simulink model "QR_Unitree_with_spine"  (R2021b)
settings: Solver=ode23t  StartTime=0.0  StopTime=10  FixedStep=1e-2  MaxStep=0.01  RelTol=1e-3  AbsTol=1e-3  EnableMultiTasking=on
values from neighbouring files (symbols this model uses):
  body_dim = [0.267 0.194 0.114]    [last_scores.mat]    (also in robotParameters.m)
  body_mass = 6.0    (= 6)    [CostOfTransport.m]    (also in last_scores.mat; robotParameters.m)
  delta_gait_front = 48    [PD_optimizedData_16Mar22_1632.mat]    (also in PD_optimizedData_16Mar22_2228_good.mat = 58; PD_optimizedData_17Mar22_1432_vel_walk_03735.mat = 56; PD_optimizedData_18Mar22_1518_right_direction.mat = 46; PD_optimizedData_18Mar22_1539.mat = 88)
  delta_gait_rear = 56    [PD_optimizedData_16Mar22_1632.mat]    (also in PD_optimizedData_16Mar22_2228_good.mat = 40; PD_optimizedData_17Mar22_1432_vel_walk_03735.mat = 6; PD_optimizedData_18Mar22_1518_right_direction.mat = 76; PD_optimizedData_18Mar22_1539.mat = 42)
  fem_der_front = [0 1.0471975512 -3.66519142919 -6.45771823238 -0.523598775598 5.41052068118 0]    [last_scores.mat]
  fem_der_rear = [0 -2.61799387799 -0.872664625997 1.2217304764 4.88692190558 1.3962634016 0]    [last_scores.mat]
  fem_motionFront = femur_motionFront    [CostFcnPDcontroll.m]    (also in CostFuncOptimizeSpine.m; last_scores.mat = [-2.12930168743 -2.33874119767 -2.26892802759 -2.12930168743; nonlinearContraints.m = deg2rad([x(1:N), x(1)]); nonlinearContraintsSpine.m = deg2rad([x(1:N), x(1)]))
  fem_motionRear = femur_motionRear    [CostFcnPDcontroll.m]    (also in CostFuncOptimizeSpine.m; last_scores.mat = [-2.09439510239 -2.12930168743 -2.16420827247 -2.19911485751; nonlinearContraints.m = deg2rad([x(2*N+1:3*N), x(2*N+1)]); nonlinearContraintsSpine.m = deg2rad([x(2*N+1:3*N), x(2*N+1)]))
  femur_height = 0.034    [last_scores.mat]    (also in robotParameters.m)
  femur_width = 0.0245    [last_scores.mat]    (also in robotParameters.m)
  gait_period = 1.2    [PD_optimizedData_16Mar22_1632.mat]    (also in PD_optimizedData_16Mar22_2228_good.mat; PD_optimizedData_17Mar22_1432_vel_walk_03735.mat; PD_optimizedData_18Mar22_1518_right_direction.mat; PD_optimizedData_18Mar22_1539.mat)
  ground = [20 2 0.1]    [last_scores.mat]    (also in robotParameters.m = [20 1.5 0.05])
  hip_mass = 0.595    [CostOfTransport.m]    (also in last_scores.mat; robotParameters.m)
  hip_radius = 0.046    [last_scores.mat]    (also in robotParameters.m)
  init_angs_F_front = deg2rad([-140 95])    [CostFcnPDcontroll.m]    (also in CostFuncOptimizeSpine.m = [q(1,1) q(2,1)]; last_scores.mat = [-2.12930168743 1.0471975512])
  init_angs_F_rear = deg2rad([-140 95])    [CostFcnPDcontroll.m]    (also in CostFuncOptimizeSpine.m = [q(1,1) q(2,1)]; last_scores.mat = [-2.09439510239 0.942477796077])
  init_angs_S_front = deg2rad([-140 95])    [CostFcnPDcontroll.m]    (also in CostFuncOptimizeSpine.m = [q(1,2) q(2,2)]; last_scores.mat = [-2.20972645936 0.894446335062])
  init_angs_S_rear = deg2rad([-140 95])    [CostFcnPDcontroll.m]    (also in CostFuncOptimizeSpine.m = [q(1,2) q(2,2)]; last_scores.mat = [-2.20954326961 0.961688146461])
  max_torque = 33.5    [last_scores.mat]    (also in robotParameters.m)
  N = (numel(x)-2)/4    [nonlinearContraints.m]    (also in nonlinearContraintsSpine.m = (numel(x)-5)/4; pampam.m = numel(params)/2)
  tib_der_front = [0 -1.74532925199 0.349065850399 0 1.57079632679 1.74532925199 0]    [last_scores.mat]
  tib_der_rear = [0 0.698131700798 -1.3962634016 3.31612557879 2.44346095279 -4.01425727959 0]    [last_scores.mat]
  tib_motionFront = tibia_motionFront    [CostFcnPDcontroll.m]    (also in CostFuncOptimizeSpine.m; last_scores.mat = [1.0471975512 0.977384381117 0.872664625997 0.977384381117 1; nonlinearContraints.m = deg2rad([x(N+1:2*N), x(N+1)]); nonlinearContraintsSpine.m = deg2rad([x(N+1:2*N), x(N+1)]))
  tib_motionRear = tibia_motionRear    [CostFcnPDcontroll.m]    (also in CostFuncOptimizeSpine.m; last_scores.mat = [0.942477796077 1.08210413624 0.733038285838 1.18682389136 1; nonlinearContraints.m = deg2rad([x(3*N+1:4*N), x(3*N+1)]); nonlinearContraintsSpine.m = deg2rad([x(3*N+1:4*N), x(3*N+1)]))
  tibia_height = 0.016    [last_scores.mat]    (also in robotParameters.m)
  tibia_width = 0.016    [last_scores.mat]    (also in robotParameters.m)
  traj_times = [0 0.2 0.4 0.6 0.8 1 1.2]    [PD_optimizedData_16Mar22_1632.mat]    (also in PD_optimizedData_16Mar22_2228_good.mat; PD_optimizedData_17Mar22_1432_vel_walk_03735.mat; PD_optimizedData_18Mar22_1518_right_direction.mat; PD_optimizedData_18Mar22_1539.mat)
  tsTraj = 0.01    [last_scores.mat]    (also in pampam.m; robotParameters.m)
undefined symbols (not defined in the file or in its folder): X, Y, Z
libraries: sm_lib x39, nesl_utility x7, robotcorelib x4, QR_library x4, simulink x4
(part 1 of 2)
settings Model: Creator=boris_1863  LastModifiedBy=yefim
settings SolverCC: MaxConsecutiveZCs=100  ZeroCrossAlgorithm=Adaptive  AlgebraicLoopSolver=TrustRegion  SolverResetMethod=Robust
settings DataIOCC: LimitDataPoints=on  MaxDataPoints=10000
settings OptimizationCC: LifeSpan=inf
settings DebuggingCC: IgnoredZcDiagnostic=none  AllowSymbolicDim=off  SFUnexpectedBacktrackingDiag=warning  SFNoUnconditionalDefaultTransitionDiag=warning  SFExecutionAtInitializationDiag=none  SFMachineParentedDataDiag=warning  ArithmeticOperatorsInVariantConditions=warning
settings HardwareCC: ProdBitPerLong=64  ProdHWDeviceType=Intel->x86-64 (Linux 64)
settings SFSimCC: SimUseLocalCustomCode=off  CustomCodeUndefinedFunction=UseInterfaceOnly
settings RTWCC: RTWUseLocalCustomCode=off
settings CodeAppCC: StateflowObjectComments=on
settings GRTTargetCC: TargetLangStandard=C89/C90 (ANSI)
settings ConfigComp: CovMetricSettings=dw  CovSaveCumulativeToWorkspaceVar=on  CovSaveSingleToWorkspaceVar=on  CovExternalEMLEnable=off  CovSFcnEnable=off
settings SimscapeCC: SimscapeLogType=all  SimscapeLogSimulationStatistics=on  SimscapeLogDataHistory=10000
settings DiagnosticsConfigSet: SimMechanicsRigidlyBoundBlock=none
settings ExplorerConfigSet: InternalSimMechanicsExplorerSettings="<ExplorerConfiguration><canonicalview>default</canonicalview><AnimationSetting><BasePlaybackSpeed>1.0</BasePlaybackSpeed><PlaybackSpeedFactor>1.0</PlaybackSpeedFactor></AnimationSetting><TilePanel><TileInfo><Tiles Columns=\"1\" Count=\"1\" Rows=\"1\"><Column Weight=\"1\"/><Row Weight=\"1\"/><Tile Height=\"1\" Width=\"1\" X=\"0\" Y=\"0\"/></Tiles></TileInfo><SceneInfo><SceneViewer><BGColor><R>1</R><G>1</G><B>1</B></BGColor><Camera><DoPerspective>off</DoPerspective><Position><X>4.34973683361565211</X><Y>-10.1418178628046327</Y><Z>0.513354401904725921</Z></Position><Center><X>4.34973683361565211</X><Y>-2.56707096496500142e-07</Y><Z>0.513354401904725921</Z></Center><Up><X>0</X><Y>-0</Y><Z>1</Z></Up><ViewLimDist>1</ViewLimDist><YLim>2.71067391231928312</YLim><XLim>5.33712410536781157</XLim></Camera></SceneViewer></SceneInfo></TilePanel><MechEditorPanel><Cameras/><GfxPanelCameraMap/><VideoCreator><PlaybackSpeedRatio>1.0</PlaybackSpeedRatio><FrameRate>30</FrameRate><VideoFormat>Motion JPEG AVI</VideoFormat><FrameSize>auto</FrameSize></VideoCreator></MechEditorPanel></ExplorerConfiguration>"

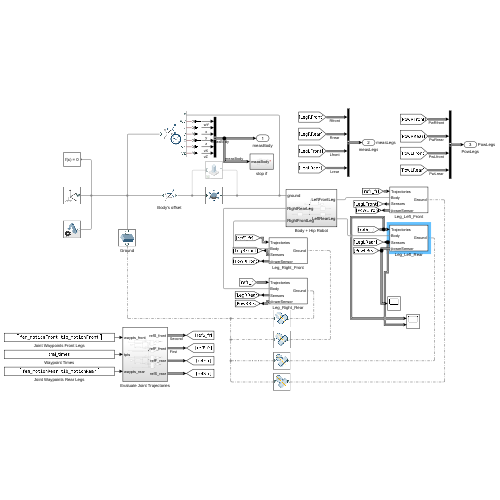
[thumbnail: Simulink's stored preview of the top-level diagram]
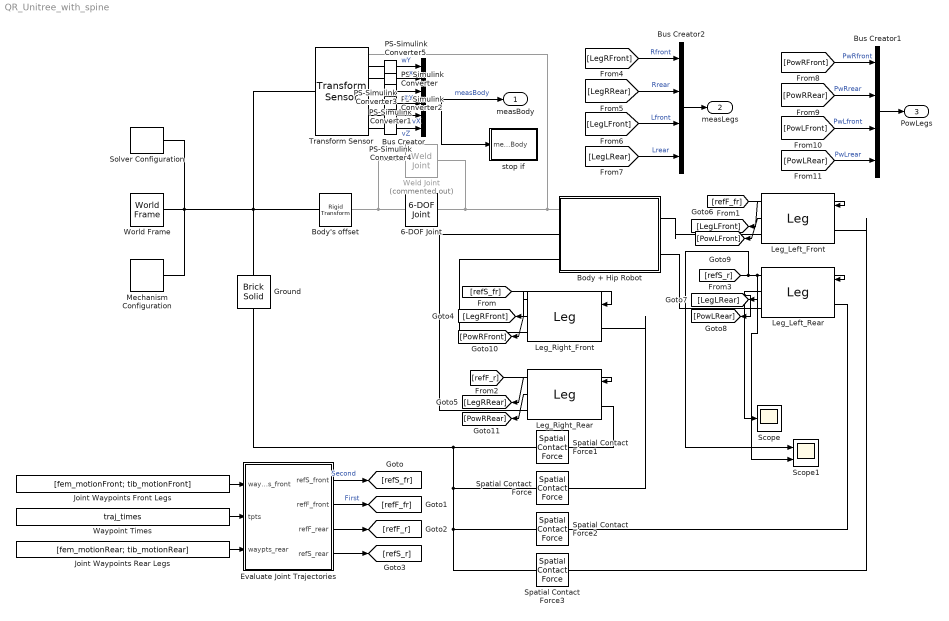
== system QR_Unitree_with_spine ==
  6-DOF Joint : sm_lib/Joints/6-DOF Joint  JointMode=Normal  SenseConstraintForce=off  SenseConstraintForceX=off  SenseConstraintForceY=off  SenseConstraintForceZ=off  SenseConstraintTorque=off  SenseConstraintTorqueX=off  SenseConstraintTorqueY=off  SenseConstraintTorqueZ=off  SenseTotalForce=off  SenseTotalForceX=off  SenseTotalForceY=off  SenseTotalForceZ=off  SenseTotalTorque=off  SenseTotalTorqueX=off  SenseTotalTorqueY=off  SenseTotalTorqueZ=off  CompositeWrenchDir=FollowerOnBase  CompositeWrenchFrame=BaseFrame  PxEquilibriumPosition=0  PxEquilibriumPositionUnits=m  PxSpringStiffness=0  PxSpringStiffnessUnits=N/m  PxDampingCoefficient=world_damping  PxDampingCoefficientUnits=N/(m/s)  PxTorqueActuationMode=NoTorque  PxMotionActuationMode=ComputedMotion  PxSensePosition=off  PxSenseVelocity=off  PxSenseAcceleration=off  PxSenseTorqueForce=off  PxSenseLowerLimitTorqueForce=off  PxSenseUpperLimitTorqueForce=off  PxLowerLimitSpecify=off  PxLowerLimitBound=-1  PxLowerLimitBoundUnits=m  PxLowerLimitStiffness=1e6  PxLowerLimitStiffnessUnits=N/m  PxLowerLimitDamping=1e3  PxLowerLimitDampingUnits=N/(m/s)  PxLowerLimitTransitionRegionWidth=1e-4  PxLowerLimitTransitionRegionWidthUnits=m  PxUpperLimitSpecify=off  PxUpperLimitBound=1  PxUpperLimitBoundUnits=m  PxUpperLimitStiffness=1e6  PxUpperLimitStiffnessUnits=N/m  PxUpperLimitDamping=1e3  PxUpperLimitDampingUnits=N/(m/s)  PxUpperLimitTransitionRegionWidth=1e-4  PxUpperLimitTransitionRegionWidthUnits=m  PxPositionTargetSpecify=off  PxPositionTargetPriority=High  PxPositionTargetValue=0  PxPositionTargetValueUnits=m  PxVelocityTargetSpecify=off  PxVelocityTargetPriority=High  PxVelocityTargetValue=0  PxVelocityTargetValueUnits=m/s  PyEquilibriumPosition=0  PyEquilibriumPositionUnits=m  PySpringStiffness=0  PySpringStiffnessUnits=N/m  PyDampingCoefficient=world_damping  PyDampingCoefficientUnits=N/(m/s)  PyTorqueActuationMode=NoTorque  PyMotionActuationMode=ComputedMotion  PySensePosition=off  PySenseVelocity=off  PySenseAcceleration=off  PySenseTorqueForce=off  PySenseLowerLimitTorqueForce=off  PySenseUpperLimitTorqueForce=off  PyLowerLimitSpecify=off  PyLowerLimitBound=-1  PyLowerLimitBoundUnits=m  PyLowerLimitStiffness=1e6  PyLowerLimitStiffnessUnits=N/m  PyLowerLimitDamping=1e3  PyLowerLimitDampingUnits=N/(m/s)  PyLowerLimitTransitionRegionWidth=1e-4  PyLowerLimitTransitionRegionWidthUnits=m  PyUpperLimitSpecify=off  PyUpperLimitBound=1  PyUpperLimitBoundUnits=m  PyUpperLimitStiffness=1e6  PyUpperLimitStiffnessUnits=N/m  PyUpperLimitDamping=1e3  PyUpperLimitDampingUnits=N/(m/s)  PyUpperLimitTransitionRegionWidth=1e-4  PyUpperLimitTransitionRegionWidthUnits=m  PyPositionTargetSpecify=off  PyPositionTargetPriority=High  PyPositionTargetValue=0  PyPositionTargetValueUnits=m  PyVelocityTargetSpecify=off  PyVelocityTargetPriority=High  PyVelocityTargetValue=0  PyVelocityTargetValueUnits=m/s  PzEquilibriumPosition=0  PzEquilibriumPositionUnits=m  PzSpringStiffness=0  PzSpringStiffnessUnits=N/m  PzDampingCoefficient=world_damping  PzDampingCoefficientUnits=N/(m/s)  PzTorqueActuationMode=NoTorque  PzMotionActuationMode=ComputedMotion  PzSensePosition=off  PzSenseVelocity=off  PzSenseAcceleration=off  PzSenseTorqueForce=off  PzSenseLowerLimitTorqueForce=off  PzSenseUpperLimitTorqueForce=off  PzLowerLimitSpecify=off  PzLowerLimitBound=-1  PzLowerLimitBoundUnits=m  PzLowerLimitStiffness=1e6  PzLowerLimitStiffnessUnits=N/m  PzLowerLimitDamping=1e3  PzLowerLimitDampingUnits=N/(m/s)  PzLowerLimitTransitionRegionWidth=1e-4  PzLowerLimitTransitionRegionWidthUnits=m  PzUpperLimitSpecify=off  PzUpperLimitBound=1  PzUpperLimitBoundUnits=m  PzUpperLimitStiffness=1e6  PzUpperLimitStiffnessUnits=N/m  PzUpperLimitDamping=1e3  PzUpperLimitDampingUnits=N/(m/s)  PzUpperLimitTransitionRegionWidth=1e-4  PzUpperLimitTransitionRegionWidthUnits=m  PzPositionTargetSpecify=off  PzPositionTargetPriority=High  PzPositionTargetValue=0  PzPositionTargetValueUnits=m  PzVelocityTargetSpecify=off  PzVelocityTargetPriority=High  PzVelocityTargetValue=0  PzVelocityTargetValueUnits=m/s  SphDefPosRotationMethod=None  SphDefPosRotationAngleUnits=deg  SphDefPosRotationStandardAxis=+Z  SphDefPosRotationAngle=0.0  SphDefPosRotationArbitraryAxis=[0 0 1]  SphDefPosFollAlignAxisA=+X  SphDefPosBaseAlignAxisA=+Y  SphDefPosFollAlignAxisB=+Y  SphDefPosBaseAlignAxisB=+Z  SphDefPosRotationSequenceAxes=FollowerAxes  SphDefPosRotationSequence=XYX  SphDefPosRotationSequenceAngles=[0 0 0]  SphDefPosRotationSequenceAnglesUnits=deg  SphDefPosRotationMatrix=[1 0 0; 0 1 0; 0 0 1]  SphEqPosRotationMethod=None  SphEqPosRotationAngleUnits=deg  SphEqPosRotationStandardAxis=+Z  SphEqPosRotationAngle=0.0  SphEqPosRotationArbitraryAxis=[0 0 1]  SphEqPosFollAlignAxisA=+X  SphEqPosBaseAlignAxisA=+Y  SphEqPosFollAlignAxisB=+Y  SphEqPosBaseAlignAxisB=+Z  SphEqPosRotationSequenceAxes=FollowerAxes  SphEqPosRotationSequence=XYX  SphEqPosRotationSequenceAngles=[0 0 0]  SphEqPosRotationSequenceAnglesUnits=deg  SphEqPosRotationMatrix=[1 0 0; 0 1 0; 0 0 1]  SphSpringStiffness=0  SphSpringStiffnessUnits=N*m/deg  SphDampingCoefficient=world_rot_damping  SphDampingCoefficientUnits=N*m/(rad/s)  SphActuateTorqueX=off  SphActuateTorqueY=off  SphActuateTorqueZ=off  SphActuateTorque=off  SphTorqueActuationMode=NoTorque  SphMotionActuationMode=ComputedMotion  SphActuationFrame=BaseFrame  SphSensePosition=off  SphSenseVelocityX=off  SphSenseVelocityY=off  SphSenseVelocityZ=off  SphSenseVelocity=off  SphSenseAccelerationX=off  SphSenseAccelerationY=off  SphSenseAccelerationZ=off  SphSenseAcceleration=off  SphSenseTorqueX=off  SphSenseTorqueY=off  SphSenseTorqueZ=off  SphSenseTorqueForce=off  SphSenseLowerLimitTorqueMag=off  SphSenseUpperLimitTorqueMag=off  SphSensingFrame=BaseFrame  SphLowerLimitSpecify=off  SphLowerLimitBound=15  SphLowerLimitBoundUnits=deg  SphLowerLimitStiffness=1e4  SphLowerLimitStiffnessUnits=N*m/deg  SphLowerLimitDamping=10  SphLowerLimitDampingUnits=N*m/(deg/s)  SphLowerLimitTransitionRegionWidth=0.1  SphLowerLimitTransitionRegionWidthUnits=deg  SphUpperLimitSpecify=off  SphUpperLimitBound=45  SphUpperLimitBoundUnits=deg  SphUpperLimitStiffness=1e4  SphUpperLimitStiffnessUnits=N*m/deg  SphUpperLimitDamping=10  SphUpperLimitDampingUnits=N*m/(deg/s)  SphUpperLimitTransitionRegionWidth=0.1  SphUpperLimitTransitionRegionWidthUnits=deg  SphPositionTargetRotationMethod=None  SphPositionTargetRotationAngleUnits=deg  SphPositionTargetRotationStandardAxis=+Z  SphPositionTargetRotationAngle=0.0  SphPositionTargetRotationArbitraryAxis=[0 0 1]  SphPositionTargetFollAlignAxisA=+X  SphPositionTargetBaseAlignAxisA=+Y  SphPositionTargetFollAlignAxisB=+Y  SphPositionTargetBaseAlignAxisB=+Z  SphPositionTargetRotationSequenceAxes=FollowerAxes  SphPositionTargetRotationSequence=XYX  SphPositionTargetRotationSequenceAngles=[0 0 0]  SphPositionTargetRotationSequenceAnglesUnits=deg  SphPositionTargetRotationMatrix=[1 0 0; 0 1 0; 0 0 1]  SphPositionTargetSpecify=off  SphPositionTargetPriority=High  SphVelocityTargetValue=[0 0 0]  SphVelocityTargetValueUnits=deg/s  SphVelocityTargetSpecify=off  SphVelocityTargetPriority=High  SphVelocityTargetInFollowerFrame=on
  Body + Hip Robot : Subsystem
  Body's offset : sm_lib/Frames and Transforms/Rigid Transform  TranslationMethod=StandardAxis  TranslationStandardOffset=z_offset  TranslationLengthUnit=m  TranslationStandardAxis=+Z  TranslationCartesianOffset=[0 0 0]  TranslationROffset=0  TranslationROffsetUnits=m  TranslationZOffset=0  TranslationZOffsetUnits=m  TranslationThetaOffset=0  TranslationThetaOffsetUnits=deg  RotationMethod=None  RotationAngleUnits=deg  RotationStandardAxis=+Z  RotationAngle=0.0  RotationArbitraryAxis=[0 0 1]  FollAlignAxisA=+X  BaseAlignAxisA=+Y  FollAlignAxisB=+Y  BaseAlignAxisB=+Z  RotationSequenceAxes=FollowerAxes  RotationSequence=XYX  RotationSequenceAngles=[0 0 0]  RotationSequenceAnglesUnits=deg  RotationMatrix=[1 0 0; 0 1 0; 0 0 1]
  Bus Creator : BusCreator  Inputs=6
  Bus Creator1 : BusCreator  Inputs=4
  Bus Creator2 : BusCreator  Inputs=4
  Evaluate Joint Trajectories : Subsystem
  Ground : sm_lib/Body Elements/Brick Solid  GraphicAmbientColor=[0.15 0.15 0.15 1.0]  BasedOnType=Density  BrickDimensions=ground  BrickDimensionUnits=m  CenterOfMass=[0 0 0]  CenterOfMassUnits=m  GraphicDiffuseColor=[0.5 0.5 0.5]  Density=1000  DensityUnits=kg/m^3  DoExposeReferenceFrame=off  GraphicEmissiveColor=[0.0 0.0 0.0 1.0]  ExportEntireGeometry=on  SerializedFrames=<Frames><Frame><Id>Frame1</Id><Value><Name>F1</Name><Origin><Source>GeometricFeature</Source><FeatureName>+z surface</FeatureName></Origin><PrimaryAxis><DefinedDirection>+Z</DefinedDirection><Source>ReferenceFrame</Source><SourceDirection>+Z</SourceDirection><FeatureName></FeatureName></PrimaryAxis><SecondaryAxis><DefinedDirection>+X</DefinedDirection><Source>ReferenceFrame</Source><SourceDirection>+X</SourceDirection><FeatureName></FeatureName></SecondaryAxis></Value></Frame></Frames>  MarkerShape=Sphere  MarkerSize=10  GraphicType=FromGeometry  InertiaType=CalculateFromGeometry  Mass=1  MassUnits=kg  MomentsOfInertia=[1 1 1]  MomentsOfInertiaUnits=kg*m^2  GraphicOpacity=1.0  ProductsOfInertia=[0 0 0]  ProductsOfInertiaUnits=kg*m^2  GraphicShininess=75  GraphicSpecularColor=[0.5 0.5 0.5 1.0]  GraphicVisPropType=SimpleVisualProperties
  Joint Waypoints Front Legs : Constant  Value=[fem_motionFront; tib_motionFront]
  Joint Waypoints Rear Legs : Constant  Value=[fem_motionRear; tib_motionRear]
  Leg_Left_Front : QR_library/Leg  femur_l=femur_length  tibia_l=tibia_length  leg_w=[femur_height, femur_width]  leg_w_t=[tibia_height, tibia_width]  qf_0=init_angs_F_front(1)  qt_0=init_angs_F_front(2)  femur_cl=[0.2 0.2 1.0]  tibia_cl=[0.6 0.6 1.0]  kp_femur=k_p_fem  ki_femur=k_i_fem  kd_femur=k_d_fem  maxFemur=max_torque  minFemur=-max_torque  kp_tibia=k_p_tib  ki_tibia=k_i_tib  kd_tibia=k_d_tib  maxTibia=max_torque  minTibia=-max_torque  pwm_freq=PWM_freq  motor_voltage=m_voltage  motor_resistance=arm_resistance  motor_inductance=arm_inductance  motor_constant=torque_c  motor_inertia=rotor_inertia  motor_damping=rotor_damping  gear_ratio=g_ratio
  Leg_Left_Rear : QR_library/Leg  femur_l=femur_length  tibia_l=tibia_length  leg_w=[femur_height, femur_width]  leg_w_t=[tibia_height, tibia_width]  qf_0=init_angs_S_rear(1)  qt_0=init_angs_S_rear(2)  femur_cl=[0.2 0.2 1.0]  tibia_cl=[0.6 0.6 1.0]  kp_femur=k_p_fem  ki_femur=k_i_fem  kd_femur=k_d_fem  maxFemur=max_torque  minFemur=-max_torque  kp_tibia=k_p_tib  ki_tibia=k_i_tib  kd_tibia=k_d_tib  maxTibia=max_torque  minTibia=-max_torque  pwm_freq=PWM_freq  motor_voltage=m_voltage  motor_resistance=arm_resistance  motor_inductance=arm_inductance  motor_constant=torque_c  motor_inertia=rotor_inertia  motor_damping=rotor_damping  gear_ratio=g_ratio
  Leg_Right_Front : QR_library/Leg  femur_l=femur_length  tibia_l=tibia_length  leg_w=[femur_height, femur_width]  leg_w_t=[tibia_height, tibia_width]  qf_0=init_angs_S_front(1)  qt_0=init_angs_S_front(2)  femur_cl=[0.2 0.2 1.0]  tibia_cl=[0.6 0.6 1.0]  kp_femur=k_p_fem  ki_femur=k_i_fem  kd_femur=k_d_fem  maxFemur=max_torque  minFemur=-max_torque  kp_tibia=k_p_tib  ki_tibia=k_i_tib  kd_tibia=k_d_tib  maxTibia=max_torque  minTibia=-max_torque  pwm_freq=PWM_freq  motor_voltage=m_voltage  motor_resistance=arm_resistance  motor_inductance=arm_inductance  motor_constant=torque_c  motor_inertia=rotor_inertia  motor_damping=rotor_damping  gear_ratio=g_ratio
  Leg_Right_Rear : QR_library/Leg  femur_l=femur_length  tibia_l=tibia_length  leg_w=[femur_height, femur_width]  leg_w_t=[tibia_height, tibia_width]  qf_0=init_angs_F_rear(1)  qt_0=init_angs_F_rear(2)  femur_cl=[0.2 0.2 1.0]  tibia_cl=[0.6 0.6 1.0]  kp_femur=k_p_fem  ki_femur=k_i_fem  kd_femur=k_d_fem  maxFemur=max_torque  minFemur=-max_torque  kp_tibia=k_p_tib  ki_tibia=k_i_tib  kd_tibia=k_d_tib  maxTibia=max_torque  minTibia=-max_torque  pwm_freq=PWM_freq  motor_voltage=m_voltage  motor_resistance=arm_resistance  motor_inductance=arm_inductance  motor_constant=torque_c  motor_inertia=rotor_inertia  motor_damping=rotor_damping  gear_ratio=g_ratio
  Mechanism Configuration : sm_lib/Utilities/Mechanism Configuration  UniformGravity=Constant  GravityVector=[0 0 -9.80665]  GravityUnits=m/s^2  LinearizationDelta=0.001  JointModeTransitionNonlinearIterations=2
  PS-Simulink Converter : nesl_utility/PS-Simulink Converter  PhysicalDomain=network_engine_domain  SubClassName=ps_output  LeftPortType=input  RightPortType=output  PseudoPeriodic=off  Frequencies=[]  Unit=m  AffineConversion=off
      settings: SourceProductBaseCode=PW,SS
  PS-Simulink Converter1 : nesl_utility/PS-Simulink Converter  PhysicalDomain=network_engine_domain  SubClassName=ps_output  LeftPortType=input  RightPortType=output  PseudoPeriodic=off  Frequencies=[]  Unit=m  AffineConversion=off
      settings: SourceProductBaseCode=PW,SS
  PS-Simulink Converter2 : nesl_utility/PS-Simulink Converter  PhysicalDomain=network_engine_domain  SubClassName=ps_output  LeftPortType=input  RightPortType=output  PseudoPeriodic=off  Frequencies=[]  Unit=m  AffineConversion=off
      settings: SourceProductBaseCode=PW,SS
  PS-Simulink Converter3 : nesl_utility/PS-Simulink Converter  PhysicalDomain=network_engine_domain  SubClassName=ps_output  LeftPortType=input  RightPortType=output  PseudoPeriodic=off  Frequencies=[]  Unit=m/s  AffineConversion=off
      settings: SourceProductBaseCode=PW,SS
  PS-Simulink Converter4 : nesl_utility/PS-Simulink Converter  PhysicalDomain=network_engine_domain  SubClassName=ps_output  LeftPortType=input  RightPortType=output  PseudoPeriodic=off  Frequencies=[]  Unit=m/s  AffineConversion=off
      settings: SourceProductBaseCode=PW,SS
  PS-Simulink Converter5 : nesl_utility/PS-Simulink Converter  PhysicalDomain=network_engine_domain  SubClassName=ps_output  LeftPortType=input  RightPortType=output  PseudoPeriodic=off  Frequencies=[]  Unit=rad/s  AffineConversion=off
      settings: SourceProductBaseCode=PW,SS
  Scope : Scope
  Scope1 : Scope  NumInputPorts=2
  Solver Configuration : nesl_utility/Solver Configuration  PhysicalDomain=network_engine_domain  SubClassName=solver  LeftPortType=input  RightPortType=generic  Tones=[]  Harmonics=[]  SimulateNoise=off  Profile=off  UseLocalSampling=off  EnableSwitchedLinearOptims=on  FrequencyDomain=off  UseCCode=off  RelTol=0.001  AbsTol=1e-06  MinStep=1e-09  ToWorkspace=off  RevertToSquareIcSolve=off  NumHomotopyIterations=100  PhasorMode=off  PhasorModeNumHarmonics=1  DoDC=off  ResidualTolerance=1e-09  UseLocalSolver=off  LocalSolverChoice=NE_BACKWARD_EULER_ADVANCER  LocalSolverSampleTime=0.001  DoFixedCost=off  MaxNonlinIter=3  MaxModeIter=2  ComputeImpulses=off  ImpulseIterations=2  LinearAlgebra=Sparse  EquationFormulation=NE_TIME_EF  DelaysMemoryBudget=1024  AutomaticFiltering=on  FilteringTimeConstant=0.001  PartitionStorageMethod=AS_NEEDED  PartitionMemoryBudget=1024  PartitionMethod=FAST
      settings: SourceProductBaseCode=PW,SS
  Spatial Contact Force{,1..3} (4 alike) : sm_lib/Forces and Torques/Spatial Contact Force  CoefficientOfDynamicFriction=dynamicFriction  CoefficientOfStaticFriction=staticFriction  SenseContactBaseRotation=off  SenseContactBaseTranslation=off  NormalDamping=cntdmp  NormalDampingUnits=N/(m/s)  SenseContactFollowerRotation=off  SenseContactFollowerTranslation=off  SenseContactSignal=off  NormalStiffness=cntstiff  NormalStiffnessUnits=N/m  FrictionalCriticalVelocity=1e-3  FrictionalCriticalVelocityUnits=m/s  ZeroCrossDetectContactStartAndEnd=off  FrictionType=SmoothStickSlip  SenseFrictionalForceMagnitude=off  SenseNormalForceMagnitude=off  NormalForceType=SmoothSpringDamper  SenseNormalVelocity=off  SenseSeparationDistance=off  SenseTangentialVelocity=off  SenseTangentialVelocityMagnitude=off  NormalTransitionRegionWidth=1e-3  NormalTransitionRegionWidthUnits=m
  Transform Sensor : sm_lib/Frames and Transforms/Transform Sensor  MeasurementFrame=World  SenseAngle=off  SenseAxis=off  SenseAngle1=off  SenseAngle2=off  SenseAngle3=off  SenseQ=off  SenseR=off  SenseOmegaX=off  SenseOmegaY=on  SenseOmegaZ=off  SenseOmega1=off  SenseOmega2=off  SenseOmega3=off  SenseQDot=off  SenseRDot=off  SenseAlphaX=off  SenseAlphaY=off  SenseAlphaZ=off  SenseAlpha1=off  SenseAlpha2=off  SenseAlpha3=off  SenseQDDot=off  SenseRDDot=off  SenseX=on  SenseY=on  SenseZ=on  SenseRad=off  SenseAzim=off  SenseDist=off  SenseInc=off  SenseXDot=on  SenseYDot=off  SenseZDot=on  SenseRadDot=off  SenseAzimDot=off  SenseDistDot=off  SenseIncDot=off  SenseXDDot=off  SenseYDDot=off  SenseZDDot=off  SenseRadDDot=off  SenseAzimDDot=off  SenseDistDDot=off  SenseIncDDot=off
  Waypoint Times : Constant  Value=traj_times
  Weld Joint : sm_lib/Joints/Weld Joint  Commented=on  JointMode=Normal  SenseConstraintForce=off  SenseConstraintForceX=off  SenseConstraintForceY=off  SenseConstraintForceZ=off  SenseConstraintTorque=off  SenseConstraintTorqueX=off  SenseConstraintTorqueY=off  SenseConstraintTorqueZ=off  SenseTotalForce=off  SenseTotalForceX=off  SenseTotalForceY=off  SenseTotalForceZ=off  SenseTotalTorque=off  SenseTotalTorqueX=off  SenseTotalTorqueY=off  SenseTotalTorqueZ=off  CompositeWrenchDir=FollowerOnBase  CompositeWrenchFrame=BaseFrame
  World Frame : sm_lib/Frames and Transforms/World Frame
  stop if : Subsystem
  measBody : Outport
  measLegs : Outport  Port=2  SignalName=measLegs
  PowLegs : Outport  Port=3  SignalName=PowLegs
  wires:
  Waypoint Times/1 -> Evaluate Joint Trajectories/2(tpts)
  Joint Waypoints Front Legs/1 -> Evaluate Joint Trajectories/1(waypts_front)
  PS-Simulink Converter/1 -> Bus Creator/2  "x"
  PS-Simulink Converter1/1 -> Bus Creator/3  "y"
  PS-Simulink Converter2/1 -> Bus Creator/4  "z"
  Bus Creator/1 -> stop if/1(measBody), measBody/1  "measBody"
  Leg_Right_Front/1 -> [LegRFront]
  Leg_Right_Rear/1 -> [LegRRear]
  Leg_Left_Front/1 -> [LegLFront]
  Leg_Left_Rear/1 -> Scope1/2, [LegLRear]
  Evaluate Joint Trajectories/1(refS_front) -> [refS_fr]  "Second"
  Evaluate Joint Trajectories/2(refF_front) -> [refF_fr]  "First"
  [refS_fr] -> Leg_Right_Front/1
  [refF_fr] -> Leg_Left_Front/1
  [refF_r] -> Leg_Right_Rear/1
  [refS_r] -> Scope1/1, Leg_Left_Rear/1
  Joint Waypoints Rear Legs/1 -> Evaluate Joint Trajectories/3(waypts_rear)
  Evaluate Joint Trajectories/3(refF_rear) -> [refF_r]
  Evaluate Joint Trajectories/4(refS_rear) -> [refS_r]
  [LegLFront] -> Bus Creator2/3  "Lfront"
  [LegRFront] -> Bus Creator2/1  "Rfront"
  Bus Creator2/1 -> measLegs/1
  [LegRRear] -> Bus Creator2/2  "Rrear"
  [LegLRear] -> Bus Creator2/4  "Lrear"
  PS-Simulink Converter3/1 -> Bus Creator/5  "vX"
  PS-Simulink Converter4/1 -> Bus Creator/6  "vZ"
  PS-Simulink Converter5/1 -> Bus Creator/1  "wY"
  Leg_Left_Rear/2 -> [PowLRear], Scope/1
  Leg_Left_Front/2 -> [PowLFront]
  Leg_Right_Front/2 -> [PowRFront]
  Leg_Right_Rear/2 -> [PowRRear]
  [PowLRear] -> Bus Creator1/4  "PwLrear"
  [PowRRear] -> Bus Creator1/2  "PwRrear"
  Bus Creator1/1 -> PowLegs/1
  [PowRFront] -> Bus Creator1/1  "PwRfront"
  [PowLFront] -> Bus Creator1/3  "PwLfront"
  connections:
  World Frame/RConn1 -- Ground/LConn1 -- Transform Sensor/LConn1 -- Body's offset/LConn1 -- Solver Configuration/RConn1 -- Mechanism Configuration/RConn1
  Weld Joint/LConn1 -- Body's offset/RConn1 -- 6-DOF Joint/LConn1
  PS-Simulink Converter/LConn1 -- Transform Sensor/RConn3
  PS-Simulink Converter1/LConn1 -- Transform Sensor/RConn4
  Transform Sensor/RConn5 -- PS-Simulink Converter2/LConn1
  Spatial Contact Force/LConn1 -- Leg_Right_Front/LConn1
  Spatial Contact Force1/LConn1 -- Leg_Right_Rear/LConn1
  Spatial Contact Force2/LConn1 -- Leg_Left_Rear/LConn1
  Spatial Contact Force3/LConn1 -- Leg_Left_Front/LConn1
  Weld Joint/RConn1 -- 6-DOF Joint/RConn1 -- Transform Sensor/RConn1 -- Body + Hip Robot/LConn1
  Leg_Right_Rear/RConn1 -- Body + Hip Robot/LConn2
  Leg_Left_Front/RConn1 -- Body + Hip Robot/RConn1
  Leg_Right_Front/RConn1 -- Body + Hip Robot/LConn3
  Body + Hip Robot/RConn2 -- Leg_Left_Rear/RConn1
  Ground/RConn1 -- Spatial Contact Force3/RConn1 -- Spatial Contact Force2/RConn1 -- Spatial Contact Force/RConn1 -- Spatial Contact Force1/RConn1
  PS-Simulink Converter3/LConn1 -- Transform Sensor/RConn6
  PS-Simulink Converter4/LConn1 -- Transform Sensor/RConn7
  PS-Simulink Converter5/LConn1 -- Transform Sensor/RConn2

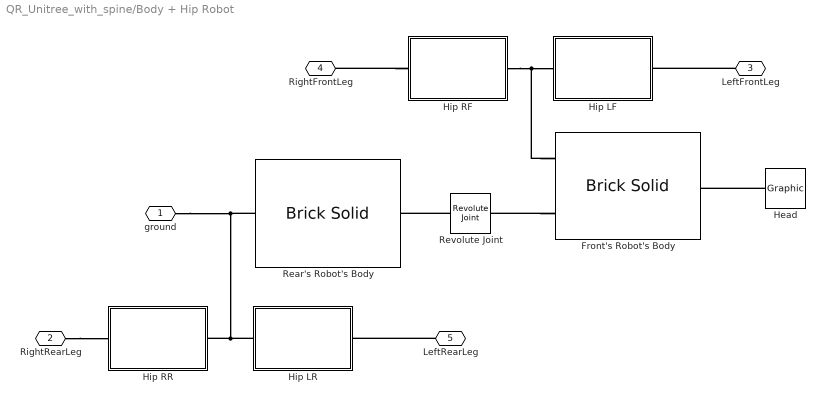
== system QR_Unitree_with_spine/Body + Hip Robot ==
  Front's Robot's Body : sm_lib/Body Elements/Brick Solid  GraphicAmbientColor=[0.15 0.15 0.15 1.0]  BasedOnType=Mass  BrickDimensions=[body_dim(1)/2 body_dim(2:3)]  BrickDimensionUnits=m  CenterOfMass=[0 0 0]  CenterOfMassUnits=m  GraphicDiffuseColor=[1.0 0.6 0.6]  Density=1000  DensityUnits=kg/m^3  DoExposeReferenceFrame=off  GraphicEmissiveColor=[0.0 0.0 0.0 1.0]  ExportEntireGeometry=off  SerializedFrames=<Frames><Frame><Id>Frame5</Id><Value><Name>world</Name><Origin><Source>GeometricFeature</Source><FeatureName>-z -x curve</FeatureName></Origin><PrimaryAxis><DefinedDirection>+Z</DefinedDirection><Source>ReferenceFrame</Source><SourceDirection>+Z</SourceDirection><FeatureName></FeatureName></PrimaryAxis><SecondaryAxis><DefinedDirection>+X</DefinedDirection><Source>ReferenceFrame</Source><SourceDirection>+X</SourceDirection><FeatureName></FeatureName></SecondaryAxis></Value></Frame><Frame><Id>Frame6</Id><Value><Name>head</Name><Origin><Source>GeometricFeature</Source><FeatureName>+z +x curve</FeatureName></Origin><PrimaryAxis><DefinedDirection>+Z</DefinedDirection><Source>ReferenceFrame</Source><SourceDirection>+Z</SourceDirection><FeatureName></FeatureName></PrimaryAxis><SecondaryAxis><DefinedDirection>+X</DefinedDirection><Source>ReferenceFrame</Source><SourceDirection>+X</SourceDirection><FeatureName></FeatureName></SecondaryAxis></Value></Frame><Frame><Id>Frame7</Id><Value><Name>spine_front</Name><Origin><Source>GeometricFeature</Source><FeatureName>-x surface</FeatureName></Origin><PrimaryAxis><DefinedDirection>+Z</DefinedDirection><Source>ReferenceFrame</Source><SourceDirection>-Y</SourceDirection><FeatureName></FeatureName></PrimaryAxis><SecondaryAxis><DefinedDirection>+X</DefinedDirection><Source>ReferenceFrame</Source><SourceDirection>+X</SourceDirection><FeatureName></FeatureName></SecondaryAxis></Value></Frame></Frames>  MarkerShape=Sphere  MarkerSize=10  GraphicType=FromGeometry  InertiaType=CalculateFromGeometry  Mass=body_mass/2  MassUnits=kg  MomentsOfInertia=[1 1 1]  MomentsOfInertiaUnits=kg*m^2  GraphicOpacity=1.0  ProductsOfInertia=[0 0 0]  ProductsOfInertiaUnits=kg*m^2  GraphicShininess=75  GraphicSpecularColor=[0.5 0.5 0.5 1.0]  GraphicVisPropType=SimpleVisualProperties
  Head : sm_lib/Body Elements/Graphic  GraphicType=Marker  MarkerShape=Frame  MarkerSize=15  GraphicVisPropType=SimpleVisualProperties  GraphicDiffuseColor=[0 0.4471 0.7412]  GraphicSpecularColor=[0.5 0.5 0.5 1.0]  GraphicAmbientColor=[0.15 0.15 0.15 1.0]  GraphicEmissiveColor=[0.0 0.0 0.0 1.0]  GraphicShininess=75  GraphicOpacity=1.0
  Hip LF : Subsystem
  Hip LR : Subsystem
  Hip RF : Subsystem
  Hip RR : Subsystem
  Rear's Robot's Body : sm_lib/Body Elements/Brick Solid  GraphicAmbientColor=[0.15 0.15 0.15 1.0]  BasedOnType=Mass  BrickDimensions=[body_dim(1)/2 body_dim(2:3)]  BrickDimensionUnits=m  CenterOfMass=[0 0 0]  CenterOfMassUnits=m  GraphicDiffuseColor=[1.0 0.6 0.6]  Density=1000  DensityUnits=kg/m^3  DoExposeReferenceFrame=off  GraphicEmissiveColor=[0.0 0.0 0.0 1.0]  ExportEntireGeometry=off  SerializedFrames=<Frames><Frame><Id>Frame5</Id><Value><Name>world</Name><Origin><Source>GeometricFeature</Source><FeatureName>-z +x curve</FeatureName></Origin><PrimaryAxis><DefinedDirection>+Z</DefinedDirection><Source>ReferenceFrame</Source><SourceDirection>+Z</SourceDirection><FeatureName></FeatureName></PrimaryAxis><SecondaryAxis><DefinedDirection>+X</DefinedDirection><Source>ReferenceFrame</Source><SourceDirection>+X</SourceDirection><FeatureName></FeatureName></SecondaryAxis></Value></Frame><Frame><Id>Frame7</Id><Value><Name>spine_rear</Name><Origin><Source>GeometricFeature</Source><FeatureName>+x surface</FeatureName></Origin><PrimaryAxis><DefinedDirection>+Z</DefinedDirection><Source>ReferenceFrame</Source><SourceDirection>-Y</SourceDirection><FeatureName></FeatureName></PrimaryAxis><SecondaryAxis><DefinedDirection>+X</DefinedDirection><Source>ReferenceFrame</Source><SourceDirection>+X</SourceDirection><FeatureName></FeatureName></SecondaryAxis></Value></Frame></Frames>  MarkerShape=Sphere  MarkerSize=10  GraphicType=FromGeometry  InertiaType=CalculateFromGeometry  Mass=body_mass/2  MassUnits=kg  MomentsOfInertia=[1 1 1]  MomentsOfInertiaUnits=kg*m^2  GraphicOpacity=1.0  ProductsOfInertia=[0 0 0]  ProductsOfInertiaUnits=kg*m^2  GraphicShininess=75  GraphicSpecularColor=[0.5 0.5 0.5 1.0]  GraphicVisPropType=SimpleVisualProperties
  Revolute Joint : sm_lib/Joints/Revolute Joint  JointMode=Normal  SenseConstraintForce=off  SenseConstraintForceX=off  SenseConstraintForceY=off  SenseConstraintForceZ=off  SenseConstraintTorque=off  SenseConstraintTorqueX=off  SenseConstraintTorqueY=off  SenseConstraintTorqueZ=off  SenseTotalForce=off  SenseTotalForceX=off  SenseTotalForceY=off  SenseTotalForceZ=off  SenseTotalTorque=off  SenseTotalTorqueX=off  SenseTotalTorqueY=off  SenseTotalTorqueZ=off  CompositeWrenchDir=FollowerOnBase  CompositeWrenchFrame=BaseFrame  EquilibriumPosition=spine_eq_pos  EquilibriumPositionUnits=rad  SpringStiffness=spine_stiffness  SpringStiffnessUnits=N*m/rad  DampingCoefficient=spine_damping  DampingCoefficientUnits=N*m/(rad/s)  TorqueActuationMode=NoTorque  MotionActuationMode=ComputedMotion  SensePosition=off  SenseVelocity=off  SenseAcceleration=off  SenseTorqueForce=off  SenseLowerLimitTorqueForce=off  SenseUpperLimitTorqueForce=off  LowerLimitSpecify=off  LowerLimitBound=spine_pos_low_limit  LowerLimitBoundUnits=rad  LowerLimitStiffness=1e4  LowerLimitStiffnessUnits=N*m/deg  LowerLimitDamping=10  LowerLimitDampingUnits=N*m/(deg/s)  LowerLimitTransitionRegionWidth=0.1  LowerLimitTransitionRegionWidthUnits=deg  UpperLimitSpecify=off  UpperLimitBound=spine_pos_up_limit  UpperLimitBoundUnits=deg  UpperLimitStiffness=1e4  UpperLimitStiffnessUnits=N*m/deg  UpperLimitDamping=10  UpperLimitDampingUnits=N*m/(deg/s)  UpperLimitTransitionRegionWidth=0.1  UpperLimitTransitionRegionWidthUnits=deg  PositionTargetSpecify=off  PositionTargetPriority=High  PositionTargetValue=0  PositionTargetValueUnits=deg  VelocityTargetSpecify=off  VelocityTargetPriority=High  VelocityTargetValue=0  VelocityTargetValueUnits=deg/s
  ground : PMIOPort  Side=Left
  RightRearLeg : PMIOPort  Port=2  Side=Left
  LeftFrontLeg : PMIOPort  Port=3  Side=Right
  RightFrontLeg : PMIOPort  Port=4  Side=Left
  LeftRearLeg : PMIOPort  Port=5  Side=Right
  connections:
  Rear's Robot's Body/LConn1 -- ground/RConn1 -- Hip LR/LConn1 -- Hip RR/LConn1
  Hip RF/RConn1 -- RightFrontLeg/RConn1
  LeftFrontLeg/RConn1 -- Hip LF/RConn1
  RightRearLeg/RConn1 -- Hip RR/RConn1
  LeftRearLeg/RConn1 -- Hip LR/RConn1
  Head/RConn1 -- Front's Robot's Body/RConn1
  Revolute Joint/LConn1 -- Rear's Robot's Body/RConn1
  Front's Robot's Body/LConn2 -- Revolute Joint/RConn1
  Hip RF/LConn1 -- Front's Robot's Body/LConn1 -- Hip LF/LConn1

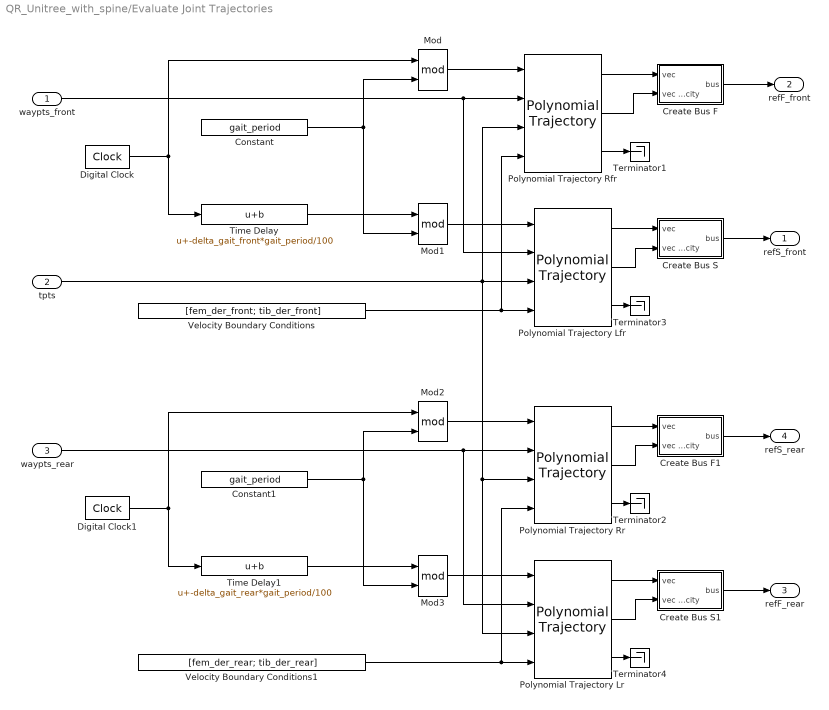
== system QR_Unitree_with_spine/Evaluate Joint Trajectories ==
  waypts_front : Inport
  tpts : Inport  Port=2
  waypts_rear : Inport  Port=3
  Constant : Constant  Value=gait_period
  Constant1 : Constant  Value=gait_period
  Create Bus F : Subsystem
  Create Bus F1 : Subsystem
  Create Bus S : Subsystem
  Create Bus S1 : Subsystem
  Digital Clock : DigitalClock  SampleTime=tsTraj
  Digital Clock1 : DigitalClock  SampleTime=tsTraj
  Mod{,1..3} (4 alike) : Math  Operator=mod  SaturateOnIntegerOverflow=on
  Polynomial Trajectory Lfr : robotcorelib/Polynomial Trajectory  WaypointSource=External  Waypoints=[ 0, 2, 1, 5, 0; -1, 3, 1, 4, 4 ]  TimePoints=[ 0, 1, 2, 3, 4 ]  TimeInterval=[ 1, 4 ]  Method=Cubic Polynomial  ParameterSource=External  VelocityBoundaryCondition=zeros( 2, 5 )  AccelerationBoundaryCondition=zeros( 2, 5 )  SimulateUsing=Interpreted execution
  Polynomial Trajectory Lr : robotcorelib/Polynomial Trajectory  WaypointSource=External  Waypoints=[ 0, 2, 1, 5, 0; -1, 3, 1, 4, 4 ]  TimePoints=[ 0, 1, 2, 3, 4 ]  TimeInterval=[ 1, 4 ]  Method=Cubic Polynomial  ParameterSource=External  VelocityBoundaryCondition=zeros( 2, 5 )  AccelerationBoundaryCondition=zeros( 2, 5 )  SimulateUsing=Interpreted execution
  Polynomial Trajectory Rfr : robotcorelib/Polynomial Trajectory  WaypointSource=External  Waypoints=[ 0, 2, 1, 5, 0; -1, 3, 1, 4, 4 ]  TimePoints=[ 0, 1, 2, 3, 4 ]  TimeInterval=[ 1, 4 ]  Method=Cubic Polynomial  ParameterSource=External  VelocityBoundaryCondition=zeros( 2, 5 )  AccelerationBoundaryCondition=zeros( 2, 5 )  SimulateUsing=Interpreted execution
  Polynomial Trajectory Rr : robotcorelib/Polynomial Trajectory  WaypointSource=External  Waypoints=[ 0, 2, 1, 5, 0; -1, 3, 1, 4, 4 ]  TimePoints=[ 0, 1, 2, 3, 4 ]  TimeInterval=[ 1, 4 ]  Method=Cubic Polynomial  ParameterSource=External  VelocityBoundaryCondition=zeros( 2, 5 )  AccelerationBoundaryCondition=zeros( 2, 5 )  SimulateUsing=Interpreted execution
  Terminator{1..4} (4 alike) : Terminator
  Time Delay : Bias  Bias=-delta_gait_front*gait_period/100
  Time Delay1 : Bias  Bias=-delta_gait_rear*gait_period/100
  Velocity Boundary Conditions : Constant  Value=[fem_der_front; tib_der_front]
  Velocity Boundary Conditions1 : Constant  Value=[fem_der_rear; tib_der_rear]
  refS_front : Outport
  refF_front : Outport  Port=2
  refF_rear : Outport  Port=3
  refS_rear : Outport  Port=4
  wires:
  Polynomial Trajectory Rfr/1 -> Create Bus F/1(vec)
  Create Bus S/1(bus) -> refS_front/1
  Create Bus F/1(bus) -> refF_front/1
  Polynomial Trajectory Lfr/1 -> Create Bus S/1(vec)
  Polynomial Trajectory Lfr/3 -> Terminator3/1
  Polynomial Trajectory Rfr/2 -> Create Bus F/2(vec velocity)
  Polynomial Trajectory Rfr/3 -> Terminator1/1
  Polynomial Trajectory Lfr/2 -> Create Bus S/2(vec velocity)
  Digital Clock/1 -> Mod/1, Time Delay/1
  waypts_front/1 -> Polynomial Trajectory Rfr/2, Polynomial Trajectory Lfr/2
  Velocity Boundary Conditions/1 -> Polynomial Trajectory Rfr/4, Polynomial Trajectory Lfr/4
  Mod/1 -> Polynomial Trajectory Rfr/1
  Mod1/1 -> Polynomial Trajectory Lfr/1
  Constant/1 -> Mod1/2, Mod/2
  Time Delay/1 -> Mod1/1
  Time Delay1/1 -> Mod3/1
  Constant1/1 -> Mod2/2, Mod3/2
  Mod3/1 -> Polynomial Trajectory Lr/1
  Mod2/1 -> Polynomial Trajectory Rr/1
  Velocity Boundary Conditions1/1 -> Polynomial Trajectory Rr/4, Polynomial Trajectory Lr/4
  tpts/1 -> Polynomial Trajectory Rfr/3, Polynomial Trajectory Lfr/3, Polynomial Trajectory Rr/3, Polynomial Trajectory Lr/3
  waypts_rear/1 -> Polynomial Trajectory Rr/2, Polynomial Trajectory Lr/2
  Digital Clock1/1 -> Time Delay1/1, Mod2/1
  Polynomial Trajectory Lr/2 -> Create Bus S1/2(vec velocity)
  Polynomial Trajectory Rr/3 -> Terminator2/1
  Polynomial Trajectory Rr/2 -> Create Bus F1/2(vec velocity)
  Polynomial Trajectory Lr/3 -> Terminator4/1
  Polynomial Trajectory Lr/1 -> Create Bus S1/1(vec)
  Create Bus F1/1(bus) -> refS_rear/1
  Create Bus S1/1(bus) -> refF_rear/1
  Polynomial Trajectory Rr/1 -> Create Bus F1/1(vec)

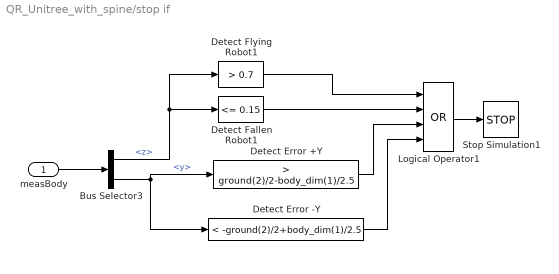
== system QR_Unitree_with_spine/stop if ==
  measBody : Inport
  Bus Selector3 : BusSelector  OutputSignals=z,y
  Detect Error +Y : simulink/Logic and Bit Operations/Compare To Constant  relop=>  const=ground(2)/2-body_dim(1)/2.5  OutDataTypeStr=boolean
  Detect Error -Y : simulink/Logic and Bit Operations/Compare To Constant  relop=<  const=-ground(2)/2+body_dim(1)/2.5  OutDataTypeStr=boolean
  Detect Fallen Robot1 : simulink/Logic and Bit Operations/Compare To Constant  relop=<=  const=0.15  OutDataTypeStr=boolean
  Detect Flying Robot1 : simulink/Logic and Bit Operations/Compare To Constant  relop=>  const=0.7  OutDataTypeStr=boolean
  Logical Operator1 : Logic  Operator=OR  Inputs=4  AllPortsSameDT=off  OutDataTypeStr=boolean
  Stop Simulation1 : Stop
  wires:
  Detect Error +Y/1 -> Logical Operator1/3
  Detect Fallen Robot1/1 -> Logical Operator1/2
  Detect Error -Y/1 -> Logical Operator1/4
  measBody/1 -> Bus Selector3/1
  Bus Selector3/1 -> Detect Fallen Robot1/1, Detect Flying Robot1/1  "<z>"
  Logical Operator1/1 -> Stop Simulation1/1
  Bus Selector3/2 -> Detect Error -Y/1, Detect Error +Y/1  "<y>"
  Detect Flying Robot1/1 -> Logical Operator1/1

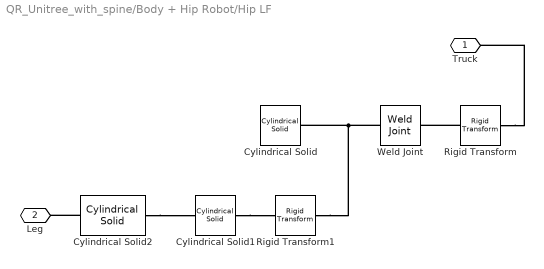
== system QR_Unitree_with_spine/Body + Hip Robot/Hip LF ==
  Cylindrical Solid : sm_lib/Body Elements/Cylindrical Solid  GraphicAmbientColor=[0.15 0.15 0.15 1.0]  BasedOnType=Density  CenterOfMass=[0 0 0]  CenterOfMassUnits=m  GraphicDiffuseColor=[0.0 0.2 0.6]  CylinderLength=hip_length  CylinderLengthUnits=m  CylinderRadius=hip_radius  CylinderRadiusUnits=m  Density=1000  DensityUnits=kg/m^3  DoExposeReferenceFrame=on  GraphicEmissiveColor=[0.0 0.0 0.0 1.0]  ExportEntireGeometry=off  SerializedFrames=<Frames/>  MarkerShape=Sphere  MarkerSize=10  GraphicType=FromGeometry  InertiaType=PointMass  Mass=hip_mass/2  MassUnits=kg  MomentsOfInertia=[1 1 1]  MomentsOfInertiaUnits=kg*m^2  GraphicOpacity=1.0  ProductsOfInertia=[0 0 0]  ProductsOfInertiaUnits=kg*m^2  GraphicShininess=75  GraphicSpecularColor=[0.5 0.5 0.5 1.0]  GraphicVisPropType=SimpleVisualProperties
  Cylindrical Solid1 : sm_lib/Body Elements/Cylindrical Solid  GraphicAmbientColor=[0.15 0.15 0.15 1.0]  BasedOnType=Density  CenterOfMass=[0 0 0]  CenterOfMassUnits=m  GraphicDiffuseColor=[0.2 0.0 0.8]  CylinderLength=hip_length  CylinderLengthUnits=m  CylinderRadius=hip_radius  CylinderRadiusUnits=m  Density=1000  DensityUnits=kg/m^3  DoExposeReferenceFrame=on  GraphicEmissiveColor=[0.0 0.0 0.0 1.0]  ExportEntireGeometry=off  SerializedFrames=<Frames><Frame><Id>Frame1</Id><Value><Name>Leg</Name><Origin><Source>GeometricFeature</Source><FeatureName>bottom surface</FeatureName></Origin><PrimaryAxis><DefinedDirection>+Z</DefinedDirection><Source>ReferenceFrame</Source><SourceDirection>+Z</SourceDirection><FeatureName></FeatureName></PrimaryAxis><SecondaryAxis><DefinedDirection>+X</DefinedDirection><Source>ReferenceFrame</Source><SourceDirection>+X</SourceDirection><FeatureName></FeatureName></SecondaryAxis></Value></Frame></Frames>  MarkerShape=Sphere  MarkerSize=10  GraphicType=FromGeometry  InertiaType=PointMass  Mass=hip_mass/2  MassUnits=kg  MomentsOfInertia=[1 1 1]  MomentsOfInertiaUnits=kg*m^2  GraphicOpacity=1.0  ProductsOfInertia=[0 0 0]  ProductsOfInertiaUnits=kg*m^2  GraphicShininess=75  GraphicSpecularColor=[0.5 0.5 0.5 1.0]  GraphicVisPropType=SimpleVisualProperties
  Cylindrical Solid2 : sm_lib/Body Elements/Cylindrical Solid  GraphicAmbientColor=[0.15 0.15 0.15 1.0]  BasedOnType=Density  CenterOfMass=[0 0 0]  CenterOfMassUnits=m  GraphicDiffuseColor=[0.2 0.2 1.0]  CylinderLength=femur_width  CylinderLengthUnits=m  CylinderRadius=hip_radius-0.01  CylinderRadiusUnits=m  Density=1000  DensityUnits=kg/m^3  DoExposeReferenceFrame=on  GraphicEmissiveColor=[0.0 0.0 0.0 1.0]  ExportEntireGeometry=off  SerializedFrames=<Frames><Frame><Id>Frame1</Id><Value><Name>hip_joint</Name><Origin><Source>GeometricFeature</Source><FeatureName>top surface</FeatureName></Origin><PrimaryAxis><DefinedDirection>+Z</DefinedDirection><Source>ReferenceFrame</Source><SourceDirection>+Z</SourceDirection><FeatureName></FeatureName></PrimaryAxis><SecondaryAxis><DefinedDirection>+X</DefinedDirection><Source>ReferenceFrame</Source><SourceDirection>+X</SourceDirection><FeatureName></FeatureName></SecondaryAxis></Value></Frame></Frames>  MarkerShape=Sphere  MarkerSize=10  GraphicType=FromGeometry  InertiaType=CalculateFromGeometry  Mass=1  MassUnits=kg  MomentsOfInertia=[1 1 1]  MomentsOfInertiaUnits=kg*m^2  GraphicOpacity=1.0  ProductsOfInertia=[0 0 0]  ProductsOfInertiaUnits=kg*m^2  GraphicShininess=75  GraphicSpecularColor=[0.5 0.5 0.5 1.0]  GraphicVisPropType=SimpleVisualProperties
  Rigid Transform : sm_lib/Frames and Transforms/Rigid Transform  TranslationMethod=Cartesian  TranslationStandardOffset=0  TranslationLengthUnit=m  TranslationStandardAxis=+Z  TranslationCartesianOffset=offset_LF  TranslationROffset=0  TranslationROffsetUnits=m  TranslationZOffset=0  TranslationZOffsetUnits=m  TranslationThetaOffset=0  TranslationThetaOffsetUnits=deg  RotationMethod=StandardAxis  RotationAngleUnits=rad  RotationStandardAxis=+X  RotationAngle=pi/2  RotationArbitraryAxis=[0 0 1]  FollAlignAxisA=+X  BaseAlignAxisA=+Y  FollAlignAxisB=+Y  BaseAlignAxisB=+Z  RotationSequenceAxes=FollowerAxes  RotationSequence=XYX  RotationSequenceAngles=[0 0 0]  RotationSequenceAnglesUnits=deg  RotationMatrix=[1 0 0; 0 1 0; 0 0 1]
  Rigid Transform1 : sm_lib/Frames and Transforms/Rigid Transform  TranslationMethod=StandardAxis  TranslationStandardOffset=hip_offset  TranslationLengthUnit=m  TranslationStandardAxis=-Z  TranslationCartesianOffset=[0 0 0]  TranslationROffset=0  TranslationROffsetUnits=m  TranslationZOffset=0  TranslationZOffsetUnits=m  TranslationThetaOffset=0  TranslationThetaOffsetUnits=deg  RotationMethod=None  RotationAngleUnits=rad  RotationStandardAxis=+X  RotationAngle=pi/2  RotationArbitraryAxis=[0 0 1]  FollAlignAxisA=+X  BaseAlignAxisA=+Y  FollAlignAxisB=+Y  BaseAlignAxisB=+Z  RotationSequenceAxes=FollowerAxes  RotationSequence=XYX  RotationSequenceAngles=[0 0 0]  RotationSequenceAnglesUnits=deg  RotationMatrix=[1 0 0; 0 1 0; 0 0 1]
  Weld Joint : sm_lib/Joints/Weld Joint  JointMode=Normal  SenseConstraintForce=off  SenseConstraintForceX=off  SenseConstraintForceY=off  SenseConstraintForceZ=off  SenseConstraintTorque=off  SenseConstraintTorqueX=off  SenseConstraintTorqueY=off  SenseConstraintTorqueZ=off  SenseTotalForce=off  SenseTotalForceX=off  SenseTotalForceY=off  SenseTotalForceZ=off  SenseTotalTorque=off  SenseTotalTorqueX=off  SenseTotalTorqueY=off  SenseTotalTorqueZ=off  CompositeWrenchDir=FollowerOnBase  CompositeWrenchFrame=BaseFrame
  Truck : PMIOPort  Side=Left
  Leg : PMIOPort  Port=2  Side=Right
  connections:
  Cylindrical Solid2/LConn1 -- Cylindrical Solid1/LConn1
  Weld Joint/RConn1 -- Cylindrical Solid/RConn1 -- Rigid Transform1/LConn1
  Rigid Transform/RConn1 -- Weld Joint/LConn1
  Rigid Transform/LConn1 -- Truck/RConn1
  Cylindrical Solid2/RConn1 -- Leg/RConn1
  Cylindrical Solid1/RConn1 -- Rigid Transform1/RConn1
